simulink model "Validacao_Sistema"  (R2012b)
settings: Solver=ode3  StartTime=0.0  StopTime=60  FixedStep=1e-4  MaxStep=1e-3
values from neighbouring files (symbols this model uses):
  denP =     [matlab.mat]
  numP =     [matlab.mat]
undefined symbols (not defined in the file or in its folder): C2t, Control_08, Control_08_Discreto, Gmf1, Gx, Planta_sistema_3
settings Model: Creator=Augusto  LastModifiedBy=Augusto

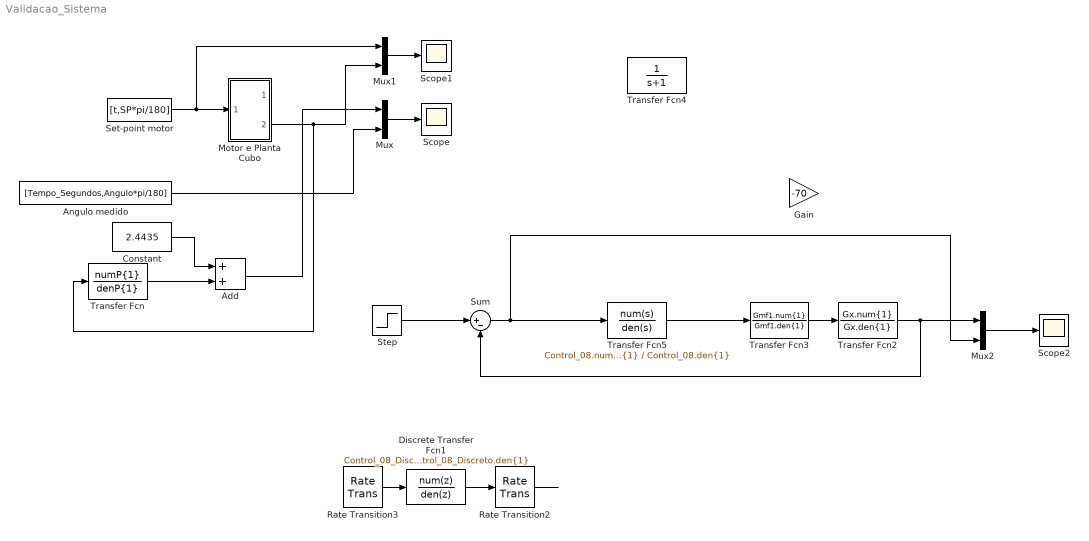
== system Validacao_Sistema ==
  Add : Sum
  Angulo medido : FromWorkspace  VariableName=[Tempo_Segundos,Angulo*pi/180]  SampleTime=0  Interpolate=off  OutputAfterFinalValue=Setting to zero
  Constant : Constant  Value=2.4435
  Discrete Transfer Fcn1 : DiscreteTransferFcn  Numerator=Control_08_Discreto.num{1}  Denominator=Control_08_Discreto.den{1}  SampleTime=0.2
  Gain : Gain  Gain=-70
  Motor e Planta Cubo : Subsystem
  Mux : Mux  Inputs=2
  Mux1 : Mux  Inputs=2
  Mux2 : Mux  Inputs=2
  Rate Transition2 : RateTransition
  Rate Transition3 : RateTransition  OutPortSampleTime=0.2
  Scope : Scope
      settings: TimeRange=140  YMin=0  YMax=6
  Scope1 : Scope
      settings: TimeRange=140  YMin=-40  YMax=40  SaveName=ScopeData2
  Scope2 : Scope
      settings: TimeRange=30  YMin=-0.4  YMax=1.4  SaveName=ScopeData3
  Set-point motor : FromWorkspace  VariableName=[t,SP*pi/180]  SampleTime=0  Interpolate=off  OutputAfterFinalValue=Setting to zero
  Step : Step  Time=0  SampleTime=0
  Sum : Sum  Inputs=|+-
  Transfer Fcn : TransferFcn  Numerator=numP{1}  Denominator=denP{1}
  Transfer Fcn2 : TransferFcn  Numerator=Gx.num{1}  Denominator=Gx.den{1}
  Transfer Fcn3 : TransferFcn  Numerator=Gmf1.num{1}  Denominator=Gmf1.den{1}
  Transfer Fcn4 : TransferFcn  Denominator=[1 1]
  Transfer Fcn5 : TransferFcn  Numerator=Control_08.num{1}  Denominator=Control_08.den{1}
  wires:
  Set-point motor/1 -> Mux1/1, Motor e Planta Cubo/1(In1)
  Angulo medido/1 -> Mux/2
  Mux/1 -> Scope/1
  Mux1/1 -> Scope1/1
  Motor e Planta Cubo/2(Omega) -> Transfer Fcn/1, Mux1/2
  Add/1 -> Mux/1
  Transfer Fcn/1 -> Add/2
  Constant/1 -> Add/1
  Step/1 -> Sum/1
  Sum/1 -> Transfer Fcn5/1, Mux2/2
  Transfer Fcn2/1 -> Mux2/1, Sum/2
  Mux2/1 -> Scope2/1
  Transfer Fcn3/1 -> Transfer Fcn2/1
  Transfer Fcn5/1 -> Transfer Fcn3/1
  Discrete Transfer Fcn1/1 -> Rate Transition2/1
  Rate Transition2/1 -> ?
  Rate Transition3/1 -> Discrete Transfer Fcn1/1

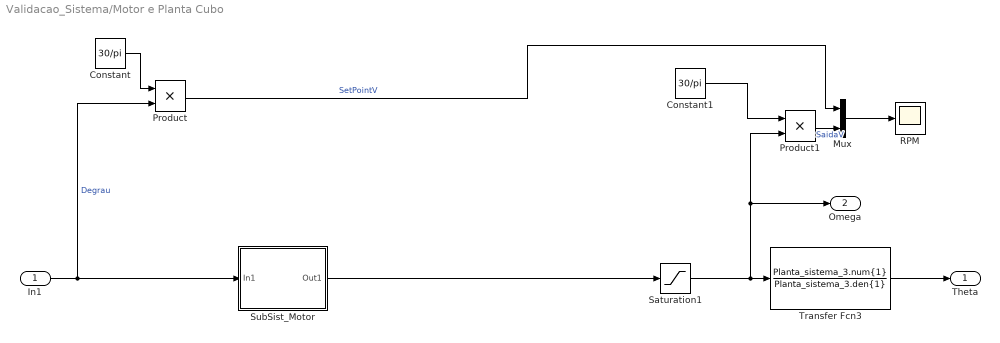
== system Validacao_Sistema/Motor e Planta Cubo ==
  In1 : Inport
  Constant : Constant  Value=30/pi
  Constant1 : Constant  Value=30/pi
  Mux : Mux  Inputs=2
  Product : Product  RndMeth=Zero
  Product1 : Product  RndMeth=Zero
  RPM : Scope
      settings: ShowLegends=on  TimeRange=50  YMin=-1000  YMax=4000
  Saturation1 : Saturate  UpperLimit=10000*pi/30  LowerLimit=-10000*pi/30
  SubSist_Motor : Subsystem
  Transfer Fcn3 : TransferFcn  Numerator=Planta_sistema_3.num{1}  Denominator=Planta_sistema_3.den{1}
  Theta : Outport
  Omega : Outport  Port=2
  wires:
  SubSist_Motor/1(Out1) -> Saturation1/1
  Transfer Fcn3/1 -> Theta/1
  Product1/1 -> Mux/2  "SaidaV"
  Saturation1/1 -> Transfer Fcn3/1, Omega/1, Product1/2
  Constant1/1 -> Product1/1
  In1/1 -> SubSist_Motor/1(In1), Product/2  "Degrau"
  Product/1 -> Mux/1  "SetPointV"
  Mux/1 -> RPM/1
  Constant/1 -> Product/1

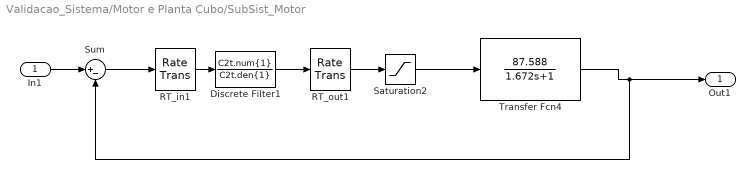
== system Validacao_Sistema/Motor e Planta Cubo/SubSist_Motor ==
  In1 : Inport
  Discrete Filter1 : DiscreteFilter  Numerator=C2t.num{1}  Denominator=C2t.den{1}  SampleTime=C2t.Ts
  RT_in1 : RateTransition  OutPortSampleTime=C2t.Ts
  RT_out1 : RateTransition
  Saturation2 : Saturate  UpperLimit=11.4  LowerLimit=-11.4
  Sum : Sum  Inputs=|+-
  Transfer Fcn4 : TransferFcn  Numerator=[87.588]  Denominator=[1.672 1]
  Out1 : Outport
  wires:
  Discrete Filter1/1 -> RT_out1/1
  RT_in1/1 -> Discrete Filter1/1
  Saturation2/1 -> Transfer Fcn4/1
  RT_out1/1 -> Saturation2/1
  In1/1 -> Sum/1
  Sum/1 -> RT_in1/1
  Transfer Fcn4/1 -> Sum/2, Out1/1
